simulink model "SMAWing_04_PID"  (R2018a)
settings: Solver=ode15s  StartTime=0.0  StopTime=5  RelTol=1e-9  AbsTol=1e-9  EnableMultiTasking=on
values from neighbouring files (symbols this model uses):
  task_params = struct    [run.m]
undefined symbols (not defined in the file or in its folder): b1, b2, Delta, I1, I2, l1, l2, m1, m2, N, params_BIAS, params_PC2, r, r1, r2
settings Model: Creator=Gianluca  LastModifiedBy=tim
settings SolverCC: AutoScaleAbsTol=off
settings DataIOCC: LimitDataPoints=on  SaveFormat=Array
settings OptimizationCC: LifeSpan=inf
settings DebuggingCC: UnderspecifiedInitializationDetection=Classic  MergeDetectMultiDrivingBlocksExec=none  SolverPrmCheckMsg=warning  StateNameClashWarn=warning  SFUnexpectedBacktrackingDiag=warning  SFNoUnconditionalDefaultTransitionDiag=warning  SFExecutionAtInitializationDiag=none
settings HardwareCC: ProdBitPerPointer=32  ProdBitPerSizeT=32  ProdBitPerPtrDiffT=32  ProdLargestAtomicFloat=None  ProdIntDivRoundTo=Undefined  ProdEndianess=Unspecified  ProdWordSize=32  ProdHWDeviceType=32-bit Generic
settings ModelReferenceCC: PropagateSignalLabelsOutOfModel=off
settings CodeAppCC: StateflowObjectComments=on
settings GRTTargetCC: TargetLangStandard=C89/C90 (ANSI)  GeneratePreprocessorConditionals=Disable all
settings ConfigComp: CovMetricSettings=dw  CovHtmlReporting=on  CovSaveCumulativeToWorkspaceVar=on  CovSaveSingleToWorkspaceVar=on  CovExternalEMLEnable=off

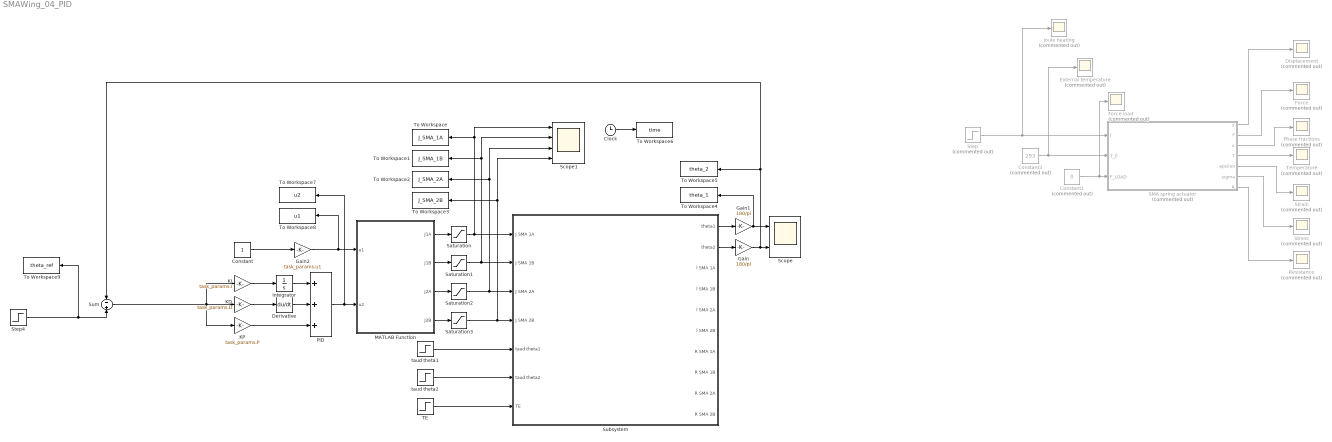
== system SMAWing_04_PID ==
  " Force load" : Scope  Commented=on
  Clock : Clock
  Constant : Constant
  Constant1 : Constant  Commented=on  Value=0
  Constant3 : Constant  Commented=on  Value=293
  Derivative : Derivative
  Displacement : Scope  Commented=on
  External temperature : Scope  Commented=on
  Force : Scope  Commented=on
  Gain : Gain  Gain=180/pi
  Gain1 : Gain  Gain=180/pi
  Gain2 : Gain  Gain=task_params.u1
  Integrator : Integrator
  Joule heating : Scope  Commented=on
  KD : Gain  Gain=task_params.D
  KI : Gain  Gain=task_params.I
  KP : Gain  Gain=task_params.P
  MATLAB Function : MATLAB Function  TreatAsAtomicUnit=on
  PID : Sum  Inputs=+++
  Phase fractions : Scope  Commented=on
  Resistance : Scope  Commented=on
  SMA spring actuator : Subsystem  Commented=on
      mask Display:
      | color('black');
      | patch(3*[-1 1 1 -1],1.1*[-1 -1 1 1],[1 1 1]);
      | patch([-1.6 -0.8],[-0.9 0.3],[0 0 0]);
      | patch([-0.8 1.2],[0.3 0.3],[0 0 0]);
      | patch([1.6 0.8],[0.9 -0.3],[0 0 0]);
      | patch([0.8 -1.2],[-0.3 -0.3],[0 0 0]);
      | disp('SMA spring');
      | 
      | color('blue');
      | port_label('input', 1, 'J [W]','texmode','on');
      | port_label('input', 2, 'T_E [K]','texmode','on');
      | port_label('input', 3, 'F_{LOAD} [N]','texmode','on');
      | 
      | color('red');
      | port_label('output', 1, 'y [m]','texmode','on');
      | port_label('output', 2, 'F [N]','texmode','on');
      | port_label('output', 3, 'x_+, x_-, x_A [-]','texmode','on');
      | port_label('output', 4, 'T [K]','texmode','on');
      | port_label('output', 5, '\epsilon [-]','texmode','on');
      | port_label('output', 6, '\sigma [Pa]','texmode','on');
      | port_label('output', 7, 'R [\Omega]','texmode','on');
  Saturation{,1..3} (4 alike) : Saturate  UpperLimit=2  LowerLimit=0
  Scope : Scope  NumInputPorts=2
  Scope1 : Scope  NumInputPorts=4
  Step : Step  Commented=on  Time=0  After=0.25  SampleTime=0
  Step4 : Step  After=50  SampleTime=0.01
  Strain : Scope  Commented=on
  Stress : Scope  Commented=on
  Subsystem : Subsystem
  Sum : Sum  Inputs=-+
  TE : Step  Time=0  Before=293  After=293  SampleTime=0
  Temperature : Scope  Commented=on
  To Workspace : ToWorkspace  VariableName=J_SMA_1A  SampleTime=0.01
  To Workspace1 : ToWorkspace  VariableName=J_SMA_1B  SampleTime=0.01
  To Workspace2 : ToWorkspace  VariableName=J_SMA_2A  SampleTime=0.01
  To Workspace3 : ToWorkspace  VariableName=J_SMA_2B  SampleTime=0.01
  To Workspace4 : ToWorkspace  VariableName=theta_1  SampleTime=0.01
  To Workspace5 : ToWorkspace  VariableName=theta_2  SampleTime=0.01
  To Workspace6 : ToWorkspace  VariableName=time  SampleTime=0.01
  To Workspace7 : ToWorkspace  VariableName=u2  SampleTime=0.01
  To Workspace8 : ToWorkspace  VariableName=u1  SampleTime=0.01
  To Workspace9 : ToWorkspace  VariableName=theta_ref  SampleTime=0.01
  taud theta1 : Step  Time=0  After=0  SampleTime=0
  taud theta2 : Step  Time=0  After=0  SampleTime=0
  wires:
  Constant3/1 -> External temperature/1, SMA spring actuator/2(T_E)
  Step/1 -> Joule heating/1, SMA spring actuator/1(J)
  Constant1/1 -> " Force load"/1, SMA spring actuator/3(F_LOAD)
  SMA spring actuator/1(y) -> Displacement/1
  SMA spring actuator/2(F) -> Force/1
  SMA spring actuator/3(x) -> Phase fractions/1
  SMA spring actuator/4(T) -> Temperature/1
  SMA spring actuator/5(epsilon) -> Strain/1
  SMA spring actuator/6(sigma) -> Stress/1
  SMA spring actuator/7(R) -> Resistance/1
  TE/1 -> Subsystem/7(TE)
  taud theta2/1 -> Subsystem/6(taud theta2)
  taud theta1/1 -> Subsystem/5(taud theta1)
  Saturation/1 -> Subsystem/1(J SMA 1A), To Workspace/1, Scope1/1
  Saturation1/1 -> Subsystem/2(J SMA 1B), To Workspace1/1, Scope1/2
  Saturation3/1 -> To Workspace3/1, Scope1/4, Subsystem/4(J SMA 2B)
  Saturation2/1 -> To Workspace2/1, Scope1/3, Subsystem/3(J SMA 2A)
  Subsystem/1(theta1) -> Gain1/1
  Subsystem/2(theta2) -> Gain/1
  Gain1/1 -> To Workspace4/1, Scope/1
  Gain/1 -> Sum/1, To Workspace5/1, Scope/2
  MATLAB Function/1(J1A) -> Saturation/1
  MATLAB Function/2(J1B) -> Saturation1/1
  MATLAB Function/3(J2A) -> Saturation2/1
  MATLAB Function/4(J2B) -> Saturation3/1
  Clock/1 -> To Workspace6/1
  Constant/1 -> Gain2/1
  Gain2/1 -> To Workspace8/1, MATLAB Function/1(u1)
  KI/1 -> Integrator/1
  KP/1 -> PID/3
  Sum/1 -> KP/1, KI/1, KD/1
  Derivative/1 -> PID/2
  KD/1 -> Derivative/1
  Integrator/1 -> PID/1
  PID/1 -> To Workspace7/1, MATLAB Function/2(u2)
  Step4/1 -> To Workspace9/1, Sum/2

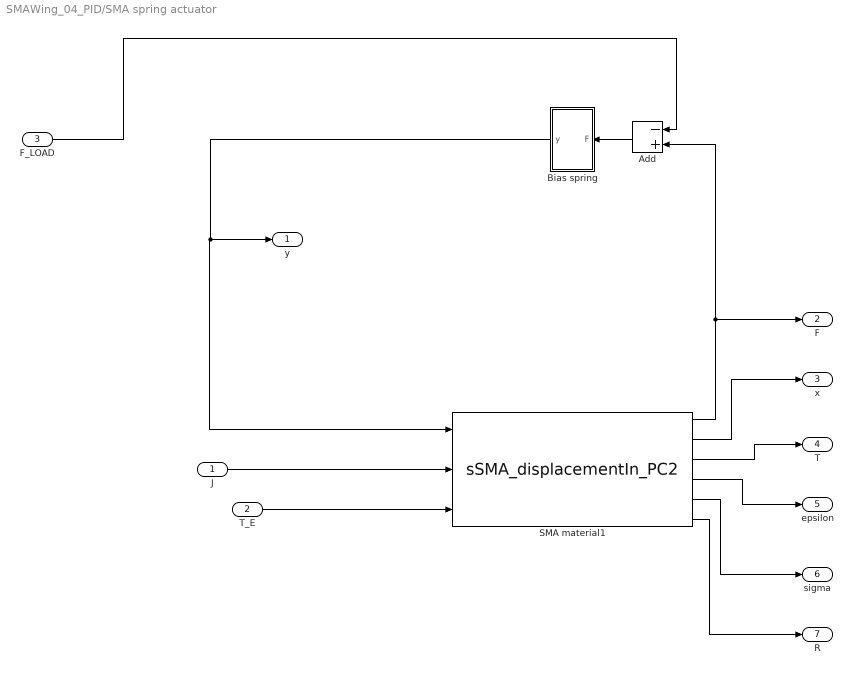
== system SMAWing_04_PID/SMA spring actuator ==
  J : Inport
  T_E : Inport  Port=2
  F_LOAD : Inport  Port=3
  Add : Sum  Inputs=-+
  Bias spring : Subsystem
  SMA material1 : M-S-Function  FunctionName=sSMA_displacementIn_PC2  Parameters=params_PC2, initConds_PC2
      mask Display:
      | color('black');
      | patch(3*[-1 1 1 -1],1.1*[-1 -1 1 1],[1 1 1]);
      | patch([-1.6 -0.8],[-0.9 0.3],[0 0 0]);
      | patch([-0.8 1.2],[0.3 0.3],[0 0 0]);
      | patch([1.6 0.8],[0.9 -0.3],[0 0 0]);
      | patch([0.8 -1.2],[-0.3 -0.3],[0 0 0]);
      | disp('SMA');
      | 
      | color('blue');
      | port_label('input', 1, 'y [m]','texmode','on');
      | port_label('input', 2, 'J [W]','texmode','on');
      | port_label('input', 3, 'T_E [K]','texmode','on');
      | 
      | color('red');
      | port_label('output', 1, 'F [N]','texmode','on');
      | port_label('output', 2, 'x_+, x_-, x_A [-]','texmode','on');
      | port_label('output', 3, 'T [K]','texmode','on');
      | port_label('output', 4, '\epsilon [-]','texmode','on');
      | port_label('output', 5, '\sigma [Pa]','texmode','on');
      | port_label('output', 6, 'R [\Omega]','texmode','on');
  y : Outport
  F : Outport  Port=2
  x : Outport  Port=3
  T : Outport  Port=4
  epsilon : Outport  Port=5
  sigma : Outport  Port=6
  R : Outport  Port=7
  wires:
  J/1 -> SMA material1/2
  T_E/1 -> SMA material1/3
  F_LOAD/1 -> Add/1
  Add/1 -> Bias spring/1(F)
  SMA material1/5 -> sigma/1
  SMA material1/1 -> F/1, Add/2
  SMA material1/2 -> x/1
  SMA material1/3 -> T/1
  SMA material1/4 -> epsilon/1
  SMA material1/6 -> R/1
  Bias spring/1(y) -> y/1, SMA material1/1

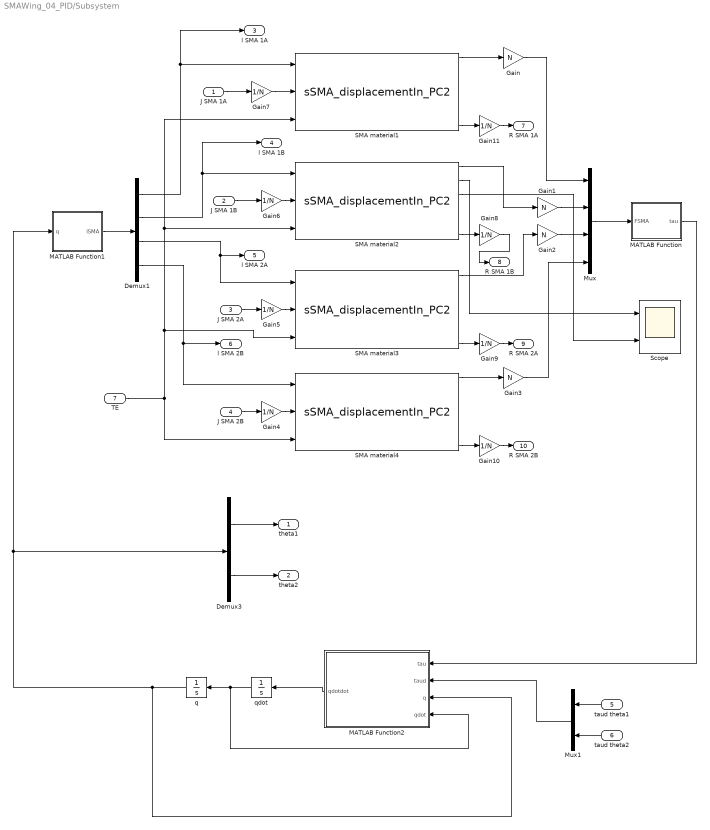
== system SMAWing_04_PID/Subsystem ==
  J SMA 1A : Inport
  J SMA 1B : Inport  Port=2
  J SMA 2A : Inport  Port=3
  J SMA 2B : Inport  Port=4
  taud theta1 : Inport  Port=5
  taud theta2 : Inport  Port=6
  TE : Inport  Port=7
  Demux1 : Demux
  Demux3 : Demux  Outputs=2
  Gain{,1..3} (4 alike) : Gain  Gain=N
  Gain{4..11} (8 alike) : Gain  Gain=1/N
  MATLAB Function : MATLAB Function  TreatAsAtomicUnit=on
  MATLAB Function1 : MATLAB Function  TreatAsAtomicUnit=on
  MATLAB Function2 : MATLAB Function  TreatAsAtomicUnit=on
  Mux : Mux
  Mux1 : Mux  Inputs=2
  SMA material{1..4} (4 alike) : M-S-Function  FunctionName=sSMA_displacementIn_PC2  Parameters=params_PC2, initConds_PC2
      mask Display:
      | color('black');
      | patch(3*[-1 1 1 -1],1.1*[-1 -1 1 1],[1 1 1]);
      | patch([-1.6 -0.8],[-0.9 0.3],[0 0 0]);
      | patch([-0.8 1.2],[0.3 0.3],[0 0 0]);
      | patch([1.6 0.8],[0.9 -0.3],[0 0 0]);
      | patch([0.8 -1.2],[-0.3 -0.3],[0 0 0]);
      | disp('SMA');
      | 
      | color('blue');
      | port_label('input', 1, 'y [m]','texmode','on');
      | port_label('input', 2, 'J [W]','texmode','on');
      | port_label('input', 3, 'T_E [K]','texmode','on');
      | 
      | color('red');
      | port_label('output', 1, 'F [N]','texmode','on');
      | port_label('output', 2, 'x_+, x_-, x_A [-]','texmode','on');
      | port_label('output', 3, 'T [K]','texmode','on');
      | port_label('output', 4, '\epsilon [-]','texmode','on');
      | port_label('output', 5, '\sigma [Pa]','texmode','on');
      | port_label('output', 6, 'R [\Omega]','texmode','on');
  Scope : Scope  NumInputPorts=2
  q : Integrator  InitialCondition=[0;0]  UpperSaturationLimit=r  LowerSaturationLimit=-r
  qdot : Integrator  InitialCondition=[0;0]
  theta1 : Outport  VectorParamsAs1DForOutWhenUnconnected=on
  theta2 : Outport  Port=2  VectorParamsAs1DForOutWhenUnconnected=on
  l SMA 1A : Outport  Port=3  VectorParamsAs1DForOutWhenUnconnected=on
  l SMA 1B : Outport  Port=4  VectorParamsAs1DForOutWhenUnconnected=on
  l SMA 2A : Outport  Port=5  VectorParamsAs1DForOutWhenUnconnected=on
  l SMA 2B : Outport  Port=6  VectorParamsAs1DForOutWhenUnconnected=on
  R SMA 1A : Outport  Port=7  VectorParamsAs1DForOutWhenUnconnected=on
  R SMA 1B : Outport  Port=8  VectorParamsAs1DForOutWhenUnconnected=on
  R SMA 2A : Outport  Port=9  VectorParamsAs1DForOutWhenUnconnected=on
  R SMA 2B : Outport  Port=10  VectorParamsAs1DForOutWhenUnconnected=on
  wires:
  q/1 -> Demux3/1, MATLAB Function1/1(q), MATLAB Function2/3(q)
  MATLAB Function/1(tau) -> MATLAB Function2/1(tau)
  MATLAB Function2/1(qdotdot) -> qdot/1
  Demux3/1 -> theta1/1
  Demux3/2 -> theta2/1
  MATLAB Function1/1(lSMA) -> Demux1/1
  qdot/1 -> MATLAB Function2/4(qdot), q/1
  taud theta2/1 -> Mux1/2
  taud theta1/1 -> Mux1/1
  Mux1/1 -> MATLAB Function2/2(taud)
  Demux1/2 -> l SMA 1B/1, SMA material2/1
  Demux1/3 -> l SMA 2A/1, SMA material3/1
  Demux1/4 -> l SMA 2B/1, SMA material4/1
  Demux1/1 -> l SMA 1A/1, SMA material1/1
  Mux/1 -> MATLAB Function/1(FSMA)
  SMA material1/1 -> Gain/1
  SMA material2/1 -> Gain1/1
  SMA material3/1 -> Gain2/1
  SMA material4/1 -> Gain3/1
  Gain/1 -> Mux/1
  Gain1/1 -> Mux/2
  Gain2/1 -> Mux/3
  Gain3/1 -> Mux/4
  J SMA 1A/1 -> Gain7/1
  J SMA 1B/1 -> Gain6/1
  J SMA 2B/1 -> Gain4/1
  Gain4/1 -> SMA material4/2
  Gain5/1 -> SMA material3/2
  J SMA 2A/1 -> Gain5/1
  Gain6/1 -> SMA material2/2
  Gain7/1 -> SMA material1/2
  TE/1 -> SMA material1/3, SMA material2/3, SMA material3/3, SMA material4/3
  SMA material2/6 -> Gain8/1
  SMA material3/6 -> Gain9/1
  SMA material4/6 -> Gain10/1
  SMA material1/6 -> Gain11/1
  Gain11/1 -> R SMA 1A/1
  Gain8/1 -> R SMA 1B/1
  Gain9/1 -> R SMA 2A/1
  Gain10/1 -> R SMA 2B/1
  SMA material2/3 -> Scope/2
  SMA material2/2 -> Scope/1

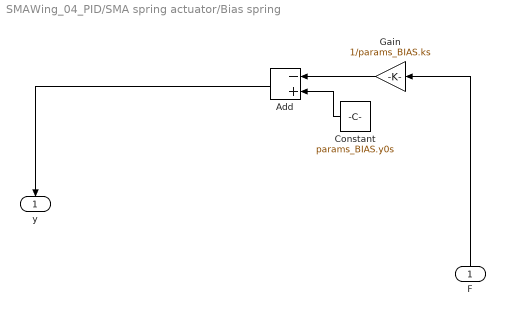
== system SMAWing_04_PID/SMA spring actuator/Bias spring ==
  F : Inport
  Add : Sum  Inputs=-+
  Constant : Constant  Value=params_BIAS.y0s
  Gain : Gain  Gain=1/params_BIAS.ks
  y : Outport
  wires:
  Add/1 -> y/1
  F/1 -> Gain/1
  Constant/1 -> Add/2
  Gain/1 -> Add/1

== matlab function SMAWing_04_PID/Subsystem/MATLAB Function1 ==
  data: lSMA output size=4; q input size=2; params_PC2 parameter; Delta parameter; r1 parameter; r2 parameter
function lSMA = fcn(q, params_PC2, Delta, r1, r2)

q1 = q(1);
q2 = q(2);
l0 = params_PC2.L0;

lSMA1A = max(l0,l0 + Delta - r1*q1);
lSMA1B = max(l0,l0 + Delta + r1*q1);
lSMA2A = max(l0,l0 + Delta - r2*q2);
lSMA2B = max(l0,l0 + Delta + r2*q2);

lSMA = [
    lSMA1A;
    lSMA1B;
    lSMA2A;
    lSMA2B
];

end

== matlab function SMAWing_04_PID/Subsystem/MATLAB Function ==
  data: FSMA input size=4; r1 parameter; r2 parameter; tau output size=2
function tau  = fcn(FSMA, r1, r2)

FSMA = reshape(FSMA, length(FSMA), 1);

J = [
    -r1 0;
    r1 0;
    0 -r2;
    0 r2
];

tau = -J'*FSMA;

== matlab function SMAWing_04_PID/Subsystem/MATLAB Function2 ==
  data: tau input size=2; taud input size=2; qdotdot output size=2; q input size=2; qdot input size=2; l2 parameter; m1 parameter; m2 parameter; I1 parameter; I2 parameter; l1 parameter; b1 parameter; b2 parameter
function qdotdot = fcn(tau, taud, q, qdot, l2, m1, m2, I1, I2, l1, b1, b2)


q1 = q(1);
q2 = q(2);
dq1 = qdot(1);
dq2 = qdot(2);

tau = reshape(tau,length(tau),1);
taud = reshape(taud,length(taud),1);

M11 = m1*l1^2/4 + I1 + m2*l1^2 + m2*l2^2/4 + m2*l1*l2*cos(q2);
M12 = m2*l2^2/4 + 1/2*m2*l1*l2*cos(q2);
M22 = m2*l2^2/4 + I2;
Mi = 1/(M11*M22 - M12^2)*[M22 -M12;-M12 M11];
C = [-m2*l1*l2*(dq1*dq2 + dq2^2/2)*sin(q2);
    1/2*m2*l1*l2*dq1^2*sin(q2)];
B = [b1 0;0 b2];

qdotdot = Mi*(-C + tau - B*qdot + taud);

== matlab function SMAWing_04_PID/MATLAB Function ==
  data: u1 input; J1A output; u2 input; J1B output; J2A output; J2B output
function [J1A, J1B, J2A, J2B] = fcn(u1, u2)
    if u1 >= 0
        J1A = abs(u1);
        J1B = 0;
    else
        J1A = 0;
        J1B = abs(u1);
    end

    if u2 >= 0
        J2A = abs(u2);
        J2B = 0;
    else
        J2A = 0;
        J2B = abs(u2);
    end
end
